simulink model "TWO_TAP_FIR"  (R2021a)
settings: Solver=VariableStepAuto  StartTime=0.0  StopTime=10.0  RelTol=1e-3
settings Model: Creator=Nimi  LastModifiedBy=Nimi

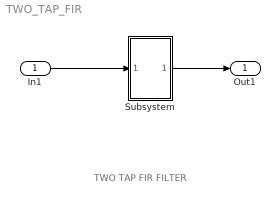
== system TWO_TAP_FIR ==
  note: TWO TAP FIR FILTER
  In1 : Inport  OutDataTypeStr=fixdt(1,8,6)
  Subsystem : Subsystem
  Out1 : Outport  OutDataTypeStr=fixdt(1,8,6)
  wires:
  In1/1 -> Subsystem/1(In1)
  Subsystem/1(Out1) -> Out1/1

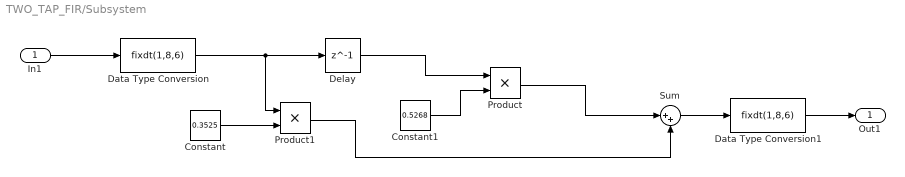
== system TWO_TAP_FIR/Subsystem ==
  In1 : Inport
  Constant : Constant  Value=0.3525  OutDataTypeStr=fixdt(1,8,6)
  Constant1 : Constant  Value=0.5268  OutDataTypeStr=fixdt(1,8,6)
  Data Type Conversion : DataTypeConversion  OutDataTypeStr=fixdt(1,8,6)
  Data Type Conversion1 : DataTypeConversion  OutDataTypeStr=fixdt(1,8,6)
  Delay : Delay  DelayLength=1
  Product : Product  OutDataTypeStr=fixdt(1,8,6)
  Product1 : Product  OutDataTypeStr=fixdt(1,8,6)
  Sum : Sum  Inputs=|++
  Out1 : Outport
  wires:
  Constant1/1 -> Product/2
  Delay/1 -> Product/1
  Product1/1 -> Sum/2
  In1/1 -> Data Type Conversion/1
  Product/1 -> Sum/1
  Sum/1 -> Data Type Conversion1/1
  Constant/1 -> Product1/2
  Data Type Conversion/1 -> Product1/1, Delay/1
  Data Type Conversion1/1 -> Out1/1
